simulink model "RC_Demo_C2000_Control_Unit"  (R2019b)
settings: Solver=FixedStepDiscrete  StartTime=0.0  StopTime=inf  FixedStep=0.01  RelTol=1e-3  EnableMultiTasking=on
undefined symbols (not defined in the file): Down, GPTRIP1SEL, GPTRIP2SEL, TZ1, TZ2, Up
libraries: c280xlib x11, canmsglib x6, dspstat3 x2, c2802xlib x2, c2837xDlib x1, c2000lib x1
settings Model: ExtModeTrigDuration=8  Creator=The MathWorks, Inc.  LastModifiedBy=bhisma
settings DataIOCC: LimitDataPoints=on  SaveFormat=Array  SaveOutput=off  SaveTime=off  ReturnWorkspaceOutputs=off
settings OptimizationCC: DefaultUnderspecifiedDataType=single  PassReuseOutputArgsAs=Individual arguments  ExpressionDepthLimit=2147483647  MaxStackSize=512  EfficientTunableParamExpr=on
settings DebuggingCC: UnderspecifiedInitializationDetection=Classic  MergeDetectMultiDrivingBlocksExec=none  SolverPrmCheckMsg=warning  MultiTaskDSMMsg=none  TasksWithSamePriorityMsg=none  ParameterPrecisionLossMsg=none  ParameterTunabilityLossMsg=error  FcnCallInpInsideContextMsg=warning  StateNameClashWarn=warning  SFUnexpectedBacktrackingDiag=warning  SFNoUnconditionalDefaultTransitionDiag=warning  SFExecutionAtInitializationDiag=none  ArithmeticOperatorsInVariantConditions=warning
settings HardwareCC: ProdBitPerChar=16  ProdBitPerInt=16  ProdBitPerPointer=32  ProdBitPerSizeT=32  ProdBitPerPtrDiffT=32  ProdLargestAtomicInteger=Integer  ProdLargestAtomicFloat=None  ProdWordSize=16  ProdLongLongMode=on  ProdHWDeviceType=Texas Instruments->C2000
settings ModelReferenceCC: PropagateSignalLabelsOutOfModel=off
settings SFSimCC: SimUseLocalCustomCode=off  CustomCodeUndefinedFunction=UseInterfaceOnly
settings RTWCC: SystemTargetFile=ert.tlc  HardwareBoard=TI Delfino F2837xD  TLCOptions=-aInlineSetEventsForThisBaseRateFcn=TLC_FALSE -aSuppressMultiTaskScheduler=TLC_FALSE -aRateBasedStepFcn=1  TemplateMakefile=ert_default_tmf  GenerateReport=on  RTWUseLocalCustomCode=off  Toolchain=Texas Instruments Code Composer Studio v6 (C2000)  IncludeHyperlinkInReport=on  LaunchReport=on  GenerateTraceInfo=on  GenerateTraceReport=on  GenerateTraceReportSl=on  GenerateTraceReportSf=on  GenerateTraceReportEml=on
settings CodeAppCC: ForceParamTrailComments=on  IgnoreCustomStorageClasses=off  OperatorAnnotations=on  SimulinkDataObjDesc=on  SFDataObjDesc=on  MATLABFcnDesc=on  InsertBlockDesc=on  StateflowObjectComments=on  MATLABSourceComments=on
settings ERTTargetCC: CodeReplacementLibrary=TI C28x
settings ConfigComp: CovMetricSettings=dw  CovHtmlReporting=on  CovSaveCumulativeToWorkspaceVar=on  CovSaveSingleToWorkspaceVar=on  CovExternalEMLEnable=off
settings TargetHardwareResources: Description=Target Hardware Resources Component

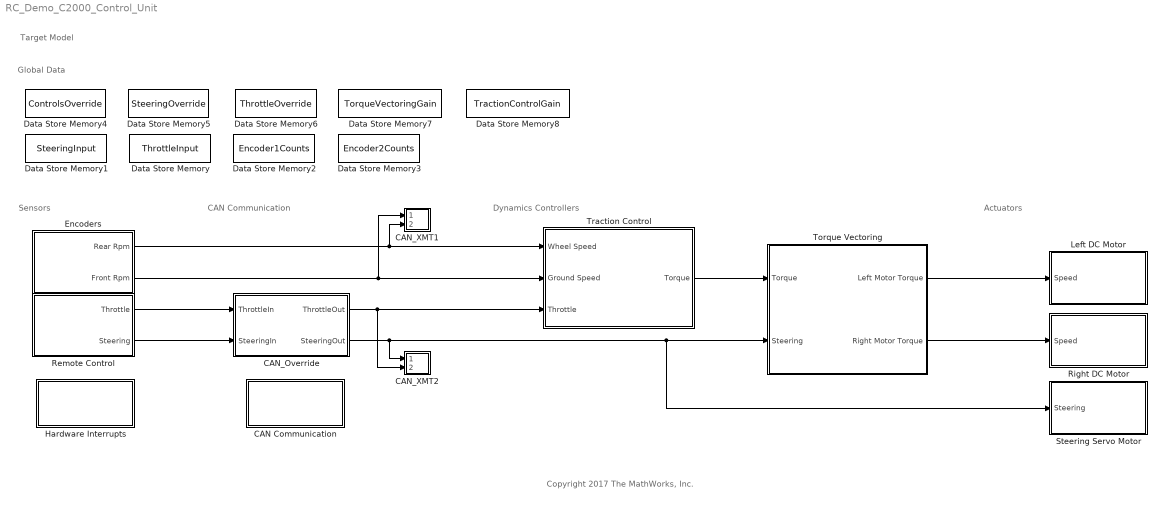
== system RC_Demo_C2000_Control_Unit ==
  note: Actuators
  note: Dynamics Controllers
  note: CAN Communication
  note: Sensors
  note: Global Data
  note: Target Model
  note: Copyright 2017 The MathWorks, Inc.
  CAN Communication : Subsystem
  CAN_Override : Subsystem
  CAN_XMT1 : Subsystem
  CAN_XMT2 : Subsystem
  Data Store Memory : DataStoreMemory  DataStoreName=ThrottleInput  ReadBeforeWriteMsg=warning  WriteAfterWriteMsg=warning  WriteAfterReadMsg=warning  ShowAdditionalParam=off
  Data Store Memory1 : DataStoreMemory  DataStoreName=SteeringInput  ReadBeforeWriteMsg=warning  WriteAfterWriteMsg=warning  WriteAfterReadMsg=warning  ShowAdditionalParam=off
  Data Store Memory2 : DataStoreMemory  DataStoreName=Encoder1Counts  ReadBeforeWriteMsg=warning  WriteAfterWriteMsg=warning  WriteAfterReadMsg=warning  ShowAdditionalParam=off  OutDataTypeStr=double
  Data Store Memory3 : DataStoreMemory  DataStoreName=Encoder2Counts  ReadBeforeWriteMsg=warning  WriteAfterWriteMsg=warning  WriteAfterReadMsg=warning  ShowAdditionalParam=off  OutDataTypeStr=double
  Data Store Memory4 : DataStoreMemory  DataStoreName=ControlsOverride  ReadBeforeWriteMsg=warning  WriteAfterWriteMsg=warning  WriteAfterReadMsg=warning  ShowAdditionalParam=off  OutDataTypeStr=int8
  Data Store Memory5 : DataStoreMemory  DataStoreName=SteeringOverride  ReadBeforeWriteMsg=warning  WriteAfterWriteMsg=warning  WriteAfterReadMsg=warning  ShowAdditionalParam=off  OutDataTypeStr=double
  Data Store Memory6 : DataStoreMemory  DataStoreName=ThrottleOverride  ReadBeforeWriteMsg=warning  WriteAfterWriteMsg=warning  WriteAfterReadMsg=warning  ShowAdditionalParam=off  OutDataTypeStr=double
  Data Store Memory7 : DataStoreMemory  DataStoreName=TorqueVectoringGain  ReadBeforeWriteMsg=warning  WriteAfterWriteMsg=warning  WriteAfterReadMsg=warning  ShowAdditionalParam=off  OutDataTypeStr=double
  Data Store Memory8 : DataStoreMemory  DataStoreName=TractionControlGain  ReadBeforeWriteMsg=warning  WriteAfterWriteMsg=warning  WriteAfterReadMsg=warning  ShowAdditionalParam=off  OutDataTypeStr=double
  Encoders : Subsystem
      mask Display:
      | pic = imread('Icons/WheelIcon.jpg');
      | pos = get_param(gcb, 'Position');
      | width  = pos(3) - pos(1);
      | height = pos(4) - pos(2);
      | x = (width - 40 - 20)/2;
      | y = (height - 40)/2;
      | image(pic,[x y 40 40]);
      | port_label('output',1,'Rear Rpm');
      | port_label('output',2,'Front Rpm');
  Hardware Interrupts : Subsystem
  Left DC Motor : Subsystem
      mask Display:
      | pic=imread('Icons/dcMotor.png');
      | image(pic,[(1-58/110)/2 (1-35/60)/2 58/110 35/60]);
      | color('blue');
      | text(0.99, 0.90, 'CAN RC Demo', 'horizontalAlignment', 'right');
  Remote Control : Subsystem
      mask Display:
      | pic = imread('Icons/SteeringIcon.png');
      | pos = get_param(gcb, 'Position');
      | width  = pos(3) - pos(1);
      | height = pos(4) - pos(2);
      | x = (width - 40 - 30)/2;
      | y = (height - 40)/2;
      | image(pic,[x y 45 40]);
      | port_label('output',1,'Throttle');
      | port_label('output',2,'Steering');
  Right DC Motor : Subsystem
      mask Display:
      | pic=imread('Icons/dcMotor.png');
      | image(pic,[(1-58/110)/2 (1-35/60)/2 58/110 35/60]);
      | color('blue');
      | text(0.99, 0.90, 'CAN RC Demo', 'horizontalAlignment', 'right');
  Steering Servo Motor : Subsystem
      mask Display:
      | pic=imread('Icons/servowrite.png');
      | image(pic,[0.32 0.23 0.35 0.53]);
      | color('blue');
      | text(0.99, 0.90, 'CAN RC Demo', 'horizontalAlignment', 'right');
  Torque Vectoring : Subsystem
      mask Display:
      | pic = imread('Icons/TVIcon.png');
      | pos = get_param(gcb, 'Position');
      | width  = pos(3) - pos(1);
      | height = pos(4) - pos(2);
      | x = (width  - 100)/2;
      | y = (height + 220)/10;
      | image(pic,[x y 80 80]);
      | port_label('output',1,'Left Motor Torque');
      | port_label('output',2,'Right Motor Torque');
      | port_label('input',1,'Torque');
      | port_label('input',2,'Steering');
  Traction Control : Subsystem
      mask Display:
      | pic = imread('Icons/TCIcon.png');
      | pos = get_param(gcb, 'Position');
      | width  = pos(3) - pos(1);
      | height = pos(4) - pos(2);
      | x = (width  - 40)/2;
      | y = (height - 80)/2;
      | image(pic,[x y 70 80]);
      | port_label('output',1,'Torque');
      | port_label('input',1,'Wheel Speed');
      | port_label('input',2,'Ground Speed');
      | port_label('input',3,'Throttle');
  wires:
  Traction Control/1(Torque) -> Torque Vectoring/1(Torque)
  CAN_Override/1(ThrottleOut) -> Traction Control/3(Throttle), CAN_XMT2/2(In2)
  CAN_Override/2(SteeringOut) -> CAN_XMT2/1(In1), Torque Vectoring/2(Steering), Steering Servo Motor/1(Steering)
  Torque Vectoring/1(Left Motor Torque) -> Left DC Motor/1(Speed)
  Torque Vectoring/2(Right Motor Torque) -> Right DC Motor/1(Speed)
  Encoders/1(Rear Rpm) -> Traction Control/1(Wheel Speed), CAN_XMT1/2(In2)
  Encoders/2(Front Rpm) -> Traction Control/2(Ground Speed), CAN_XMT1/1(In1)
  Remote Control/1(Throttle) -> CAN_Override/1(ThrottleIn)
  Remote Control/2(Steering) -> CAN_Override/2(SteeringIn)

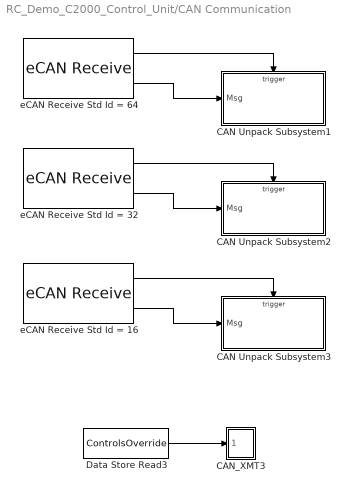
== system RC_Demo_C2000_Control_Unit/CAN Communication ==
  CAN Unpack Subsystem1 : Subsystem  TreatAsAtomicUnit=on
  CAN Unpack Subsystem2 : Subsystem  TreatAsAtomicUnit=on
  CAN Unpack Subsystem3 : Subsystem  TreatAsAtomicUnit=on
  CAN_XMT3 : Subsystem
  Data Store Read3 : DataStoreRead  DataStoreName=ControlsOverride
  eCAN Receive Std Id = 16 : c280xlib/eCAN Receive  chipFamily=C280x  useModule=eCAN_B  mailboxNo=17  messageID=16  messageType=Standard (11-bit identifier)  sampleTime=0.01  dataType=CAN_MESSAGE_TYPE  initValue=0  outputMessageLength=off  outputMessageTimeStamp=off  postInterrupt=off  interruptLine=0
      settings: SourceProductName=Embedded Coder Support Package for Texas Instruments C2000 Processors  SourceProductBaseCode=TIC2000
  eCAN Receive Std Id = 32 : c280xlib/eCAN Receive  chipFamily=C280x  useModule=eCAN_B  mailboxNo=16  messageID=32  messageType=Standard (11-bit identifier)  sampleTime=0.01  dataType=CAN_MESSAGE_TYPE  initValue=0  outputMessageLength=off  outputMessageTimeStamp=off  postInterrupt=off  interruptLine=0
      settings: SourceProductName=Embedded Coder Support Package for Texas Instruments C2000 Processors  SourceProductBaseCode=TIC2000
  eCAN Receive Std Id = 64 : c280xlib/eCAN Receive  chipFamily=C280x  useModule=eCAN_B  mailboxNo=15  messageID=64  messageType=Standard (11-bit identifier)  sampleTime=0.01  dataType=CAN_MESSAGE_TYPE  initValue=0  outputMessageLength=off  outputMessageTimeStamp=off  postInterrupt=off  interruptLine=0
      settings: SourceProductName=Embedded Coder Support Package for Texas Instruments C2000 Processors  SourceProductBaseCode=TIC2000
  wires:
  eCAN Receive Std Id = 64/1 -> CAN Unpack Subsystem1/Trigger
  eCAN Receive Std Id = 64/2 -> CAN Unpack Subsystem1/1(Msg)
  eCAN Receive Std Id = 32/1 -> CAN Unpack Subsystem2/Trigger
  eCAN Receive Std Id = 32/2 -> CAN Unpack Subsystem2/1(Msg)
  Data Store Read3/1 -> CAN_XMT3/1(In1)
  eCAN Receive Std Id = 16/2 -> CAN Unpack Subsystem3/1(Msg)
  eCAN Receive Std Id = 16/1 -> CAN Unpack Subsystem3/Trigger

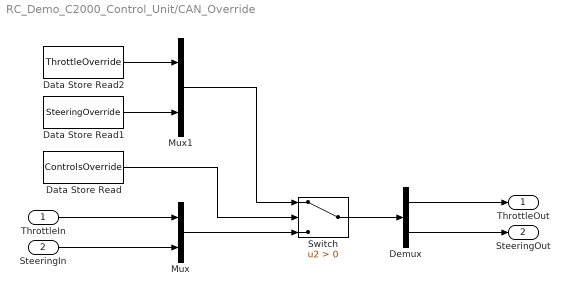
== system RC_Demo_C2000_Control_Unit/CAN_Override ==
  ThrottleIn : Inport
  SteeringIn : Inport  Port=2
  Data Store Read : DataStoreRead  DataStoreName=ControlsOverride
  Data Store Read1 : DataStoreRead  DataStoreName=SteeringOverride
  Data Store Read2 : DataStoreRead  DataStoreName=ThrottleOverride
  Demux : Demux  Outputs=2
  Mux : Mux  Inputs=2
  Mux1 : Mux  Inputs=2
  Switch : Switch  Criteria=u2 > Threshold
  ThrottleOut : Outport
  SteeringOut : Outport  Port=2
  wires:
  Data Store Read/1 -> Switch/2
  Mux1/1 -> Switch/1
  Mux/1 -> Switch/3
  Switch/1 -> Demux/1
  SteeringIn/1 -> Mux/2
  ThrottleIn/1 -> Mux/1
  Demux/1 -> ThrottleOut/1
  Demux/2 -> SteeringOut/1
  Data Store Read1/1 -> Mux1/2
  Data Store Read2/1 -> Mux1/1

== system RC_Demo_C2000_Control_Unit/CAN_XMT1 ==
  In1 : Inport
  In2 : Inport  Port=2
  CAN Pack1 : canmsglib/CAN Pack  CANdbFile=C:\Users\josea\Desktop\C2000\CAN\Vector\RCDemo.dbc  MsgList=WheelSpeeds  MsgName=WheelSpeeds  MsgIDType=Standard (11-bit identifier)  MsgIdentifier=48  MsgLength=8  SignalInfo=FrontWheelSpeed$24$32$2$3$1$0$1$0$-3.400000e+38$3.400000e+38$#RearWheelSpeed$56$32$2$3$1$0$1$0$-3.400000e+38$3.400000e+38$#  NSignals=2  StartBits=str2num('[int32(24);int32(56)]')  SignalSizes=str2num('[int32(32);int32(32)]')  ByteOrders=str2num('[int32(2);int32(2)]')  DataTypes=str2num('[int32(3);int32(3)]')  MultiplexTypes=str2num('[int32(1);int32(1)]')  MultiplexValues=str2num('[double(0);double(0)]')  Factors=str2num('[double(1);double(1)]')  Offsets=str2num('[double(0);double(0)]')  Minimums=str2num('[double(-3.400000e+38);double(-3.400000e+38)]')  Maximums=str2num('[double(3.400000e+38);double(3.400000e+38)]')  Remote=off  ApplyMinMax=off
      settings: SourceProductName=Simulink Real-Time  DataFormat=CANdb specified signals
  eCAN Transmit1 : c280xlib/eCAN Transmit  chipFamily=C280x  useModule=eCAN_B  mailboxNo=0  messageID=48  messageType=Standard (11-bit identifier)  enableBlockingMode=off  postInterrupt=off  interruptLine=0
      settings: SourceProductName=Embedded Coder Support Package for Texas Instruments C2000 Processors  SourceProductBaseCode=TIC2000
  wires:
  CAN Pack1/1 -> eCAN Transmit1/1
  In1/1 -> CAN Pack1/1
  In2/1 -> CAN Pack1/2

== system RC_Demo_C2000_Control_Unit/CAN_XMT2 ==
  In1 : Inport
  In2 : Inport  Port=2
  CAN Pack2 : canmsglib/CAN Pack  CANdbFile=C:\Users\josea\Desktop\C2000\CAN\Vector\RCDemo.dbc  MsgList=DriverControlsFromCar  MsgName=DriverControlsFromCar  MsgIDType=Standard (11-bit identifier)  MsgIdentifier=33  MsgLength=8  SignalInfo=SteeringInput$32$32$1$3$1$0$1$0$-3.400000e+38$3.400000e+38$#ThrottleInput$0$32$1$3$1$0$1$0$-3.400000e+38$3.400000e+38$#  NSignals=2  StartBits=str2num('[int32(32);int32(0)]')  SignalSizes=str2num('[int32(32);int32(32)]')  ByteOrders=str2num('[int32(1);int32(1)]')  DataTypes=str2num('[int32(3);int32(3)]')  MultiplexTypes=str2num('[int32(1);int32(1)]')  MultiplexValues=str2num('[double(0);double(0)]')  Factors=str2num('[double(1);double(1)]')  Offsets=str2num('[double(0);double(0)]')  Minimums=str2num('[double(-3.400000e+38);double(-3.400000e+38)]')  Maximums=str2num('[double(3.400000e+38);double(3.400000e+38)]')  Remote=off  ApplyMinMax=off
      settings: SourceProductName=Simulink Real-Time  DataFormat=CANdb specified signals
  eCAN Transmit2 : c280xlib/eCAN Transmit  chipFamily=C280x  useModule=eCAN_B  mailboxNo=1  messageID=33  messageType=Standard (11-bit identifier)  enableBlockingMode=off  postInterrupt=off  interruptLine=0
      settings: SourceProductName=Embedded Coder Support Package for Texas Instruments C2000 Processors  SourceProductBaseCode=TIC2000
  wires:
  CAN Pack2/1 -> eCAN Transmit2/1
  In2/1 -> CAN Pack2/2
  In1/1 -> CAN Pack2/1

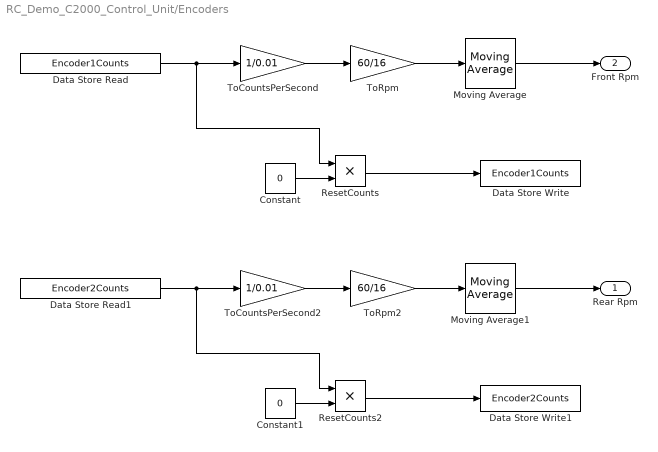
== system RC_Demo_C2000_Control_Unit/Encoders ==
  Constant : Constant  Value=0
  Constant1 : Constant  Value=0
  Data Store Read : DataStoreRead  Priority=1  DataStoreName=Encoder1Counts
  Data Store Read1 : DataStoreRead  Priority=1  DataStoreName=Encoder2Counts
  Data Store Write : DataStoreWrite  DataStoreName=Encoder1Counts
  Data Store Write1 : DataStoreWrite  DataStoreName=Encoder2Counts
  Moving Average : dspstat3/Moving Average  Method=Sliding window  SpecifyWindowLength=on  WindowLength=10  ForgettingFactor=0.9  SimulateUsing=Code generation
  Moving Average1 : dspstat3/Moving Average  Method=Sliding window  SpecifyWindowLength=on  WindowLength=10  ForgettingFactor=0.9  SimulateUsing=Code generation
  ResetCounts : Product  Inputs=**
  ResetCounts2 : Product  Inputs=**
  ToCountsPerSecond : Gain  Gain=1/0.01
  ToCountsPerSecond2 : Gain  Gain=1/0.01
  ToRpm : Gain  Gain=60/16
  ToRpm2 : Gain  Gain=60/16
  Rear Rpm : Outport
  Front Rpm : Outport  Port=2
  wires:
  Moving Average1/1 -> Rear Rpm/1
  Data Store Read1/1 -> ResetCounts2/1, ToCountsPerSecond2/1
  ToCountsPerSecond2/1 -> ToRpm2/1
  ToRpm2/1 -> Moving Average1/1
  Constant1/1 -> ResetCounts2/2
  ResetCounts2/1 -> Data Store Write1/1
  ResetCounts/1 -> Data Store Write/1
  Constant/1 -> ResetCounts/2
  ToRpm/1 -> Moving Average/1
  ToCountsPerSecond/1 -> ToRpm/1
  Data Store Read/1 -> ToCountsPerSecond/1, ResetCounts/1
  Moving Average/1 -> Front Rpm/1

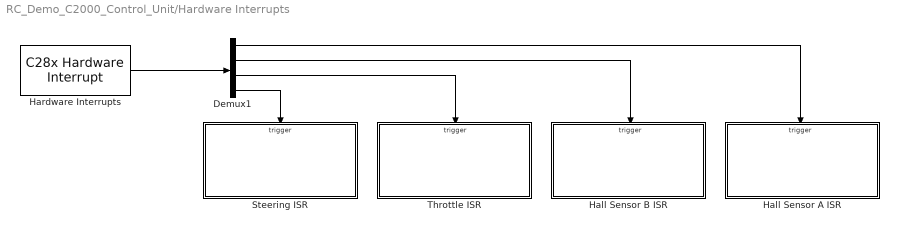
== system RC_Demo_C2000_Control_Unit/Hardware Interrupts ==
  Demux1 : Demux
  Hall Sensor A ISR : Subsystem  TreatAsAtomicUnit=on
  Hall Sensor B ISR : Subsystem  TreatAsAtomicUnit=on
  Hardware Interrupts : c2000lib/Scheduling/C28x Hardware Interrupt  irqnumbers=[4 4 4 4]  pienumbers=[1 2 3 4]  irqpriorities=[25 25 2 2]  irqpreempts=[1 1 0 0]  showinput=off  dspchiptype=C280X
      settings: SourceProductName=Embedded Coder Support Package for Texas Instruments C2000 Processors  SourceProductBaseCode=TIC2000
  Steering ISR : Subsystem  TreatAsAtomicUnit=on
  Throttle ISR : Subsystem  TreatAsAtomicUnit=on
  wires:
  Hardware Interrupts/1 -> Demux1/1
  Demux1/1 -> Hall Sensor A ISR/Trigger
  Demux1/4 -> Steering ISR/Trigger
  Demux1/3 -> Throttle ISR/Trigger
  Demux1/2 -> Hall Sensor B ISR/Trigger

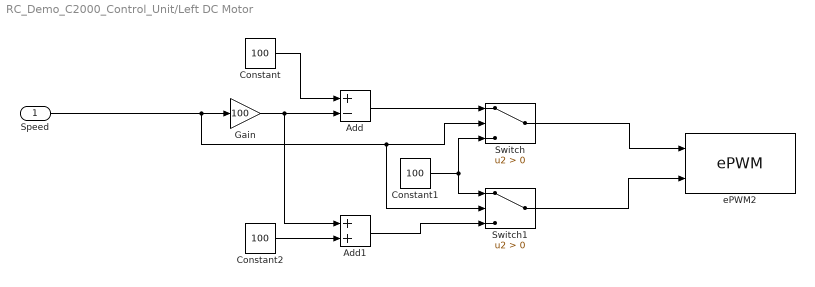
== system RC_Demo_C2000_Control_Unit/Left DC Motor ==
  Speed : Inport
  Add : Sum  Inputs=+-
  Add1 : Sum
  Constant : Constant  Value=100
  Constant1 : Constant  Value=100
  Constant2 : Constant  Value=100
  Gain : Gain  Gain=100
  Switch : Switch  Criteria=u2 > Threshold
  Switch1 : Switch  Criteria=u2 > Threshold
  ePWM2 : c2802xlib/ePWM  useModule=ePWM2  ePWMxLINKTBPRD=Not Linked  periodUnits=Clock cycles  timerSource=Specify via dialog  timerPeriod_clk=4000  timerPeriod_sec=0.02  tbshadow=Counter equals to zero  countingMode=Up-Down  phaseActiveEnable=Disable  phaseDirection=Count down after sync  phaseActive=0  synchronizationEnable=off  dcaevt1Sync=off  dcbevt1Sync=off  synchronizationOption=Disable  clockPrescale=1  HSclockPrescale=1  enswap=off  ePWMxAStatus=on  ePWMxAactionLogic1=Do nothing  ePWMxAactionLogic2=Do nothing  ePWMxAactionLogic3=Set  ePWMxAactionLogic4=Clear  ePWMxAactionLogic5=Do nothing  ePWMxAactionLogic6=Do nothing  ePWMxALoadMode=Load on counter equals to zero (CTR=Zero)  ePWMxACSFenable=off  ePWMxACSFvalue=Forcing disable  ePWMxASFreload=Zero  ePWMxBStatus=on  ePWMxBactionLogic1=Do nothing  ePWMxBactionLogic2=Do nothing  ePWMxBactionLogic3=Do nothing  ePWMxBactionLogic4=Do nothing  ePWMxBactionLogic5=Set  ePWMxBactionLogic6=Clear  ePWMxBLoadMode=Load on counter equals to zero (CTR=Zero)  ePWMxBCSFenable=off  ePWMxBCSFvalue=Forcing disable  ePWMxBSFreload=Zero  ePWNxBOutWay=off  ePWMxLINKCMPA=Not Linked  CMPAUnits=Percentages  CMPASource=Input port  CMPAValue_per=0  CMPAValue_clk=5000  enCMPAshadow=Counter equals to zero  ePWMxLINKCMPB=Not Linked  CMPBUnits=Percentages  CMPBSource=Input port  CMPBValue_per=0  CMPBValue_clk=0  enCMPBshadow=Counter equals to zero  ePWMxLINKCMPC=Not Linked  CMPCUnits=Clock cycles  CMPCSource=Specify via dialog  CMPCValue_per=50  CMPCValue_clk=0  enCMPCshadow=Counter equals to zero  ePWMxLINKCMPD=Not Linked  CMPDUnits=Clock cycles  CMPDSource=Specify via dialog  CMPDValue_per=50  CMPDValue_clk=0  enCMPDshadow=Counter equals to zero  enableDBePWMxA=off  enableDBePWMxB=off  enhalfcycle=off  DBpolarity=Active high (AH)  DBedgeDelay=Positive  DBSource_ePWMxA=ePWMxA  DBSource_ePWMxB=ePWMxA  DBperiodSource=Specify via dialog  REDperiod=0  FEDperiod=0  adcstartModuleA=on  adcrequestEventA=First event  adcstartEventA=Digital Compare Module A Event 1 start of conversion (DCAEVT1.soc)  adcstartEventA_type2=Counter equals to period (CTR=PRD)  adcstartModuleB=on  adcrequestEventB=First event  adcstartEventB=Counter equals to zero (CTR=Zero)  adcstartEventB_type2=Counter equals to zero (CTR=Zero)  intEn=off  intPrd=First event  intSel=Counter equals to zero (CTR=Zero)  intSel_type2=Counter equals to zero (CTR=Zero)  hrpe=off  enHRPWM=off  HRPWM_LoadMode=Counter equals to period (CTR=PRD)  HRPWM_CTLMode=Duty or Period control mode  HRPWM_EDGMode=Both edge  hrpeb=off  enHRPWMB=off  HRPWM_LoadModeB=Counter equals to zero (CTR=ZERO)  HRPWM_CTLModeB=Duty or Period control mode  HRPWM_EDGModeB=Both edge  enSFO=on  enautoconv=on  chopperEnable=off  chopperFrequency=1  chopperFirstwidth=1  chopperDuty=12.5%  tripZonesource=Specify via dialog  tzselOSHT1=off  tzselOSHT2=off  tzselOSHT3=off  tzselOSHDCAEV1=off  tzselOSHDCBEV1=off  tzselCBC1=off  tzselCBC2=off  tzselCBC3=off  tzselCBCDCAEV2=off  tzselCBCDCBEV2=off  tzselOSHT4=off  tzselOSHT5=off  tzselOSHT6=off  tzselCBC4=off  tzselCBC5=off  tzselCBC6=off  enTzOstIntr=off  enTzCbcIntr=off  enTzDCAEVT1Intr=off  enTzDCAEVT2Intr=off  enTzDCBEVT1Intr=off  enTzDCBEVT2Intr=off  ePWMxAforced=No action  ePWMxBforced=No action  DCAEVT1forced=No action  DCBEVT1forced=No action  DCAEVT2forced=No action  DCBEVT2forced=No action  dcah=Trip Zone 1 input (TZ1)  dcal=Trip Zone 2 input (TZ2)  dcbh=Trip Zone 1 input (TZ1)  dcbl=Trip Zone 2 input (TZ2)  dcah_type2=GPTRIP1SEL/(TZ1)  dcal_type2=GPTRIP2SEL/(TZ2)  dcbh_type2=GPTRIP1SEL/(TZ1)  dcbl_type2=GPTRIP2SEL/(TZ2)  gendcaevt1=Event disabled  gendcaevt2=Event disabled  gendcbevt1=Event disabled  gendcbevt2=Event disabled  dcaevt1src=DCAEVT1 with sync  dcaevt2src=DCAEVT2 with sync  dcbevt1src=DCBEVT1 with sync  dcbevt2src=DCBEVT2 with sync  pulsesel=Counter equals to zero (CTR=Zero)  blankinv=off  blankoffset=0  blankwidth=0  evsrcsel=Filtered version of DCAEVT1 (DCAEVT1FILT)  encape=off  PwmType=C2000_Type4
      settings: SourceProductName=Embedded Coder Support Package for Texas Instruments C2000 Processors
  wires:
  Switch/1 -> ePWM2/1
  Constant2/1 -> Add1/2
  Add/1 -> Switch/1
  Add1/1 -> Switch1/3
  Constant1/1 -> Switch/3, Switch1/1
  Constant/1 -> Add/1
  Gain/1 -> Add1/1, Add/2
  Speed/1 -> Switch1/2, Switch/2, Gain/1
  Switch1/1 -> ePWM2/2

== system RC_Demo_C2000_Control_Unit/Remote Control ==
  Data Store Read : DataStoreRead  DataStoreName=ThrottleInput
  Data Store Read1 : DataStoreRead  DataStoreName=SteeringInput
  Throttle : Outport
  Steering : Outport  Port=2
  wires:
  Data Store Read/1 -> Throttle/1
  Data Store Read1/1 -> Steering/1

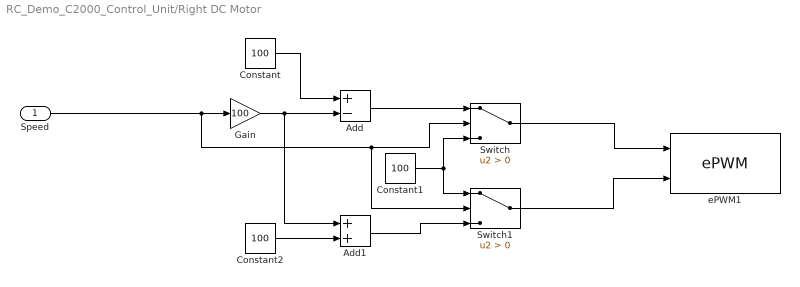
== system RC_Demo_C2000_Control_Unit/Right DC Motor ==
  Speed : Inport
  Add : Sum  Inputs=+-
  Add1 : Sum
  Constant : Constant  Value=100
  Constant1 : Constant  Value=100
  Constant2 : Constant  Value=100
  Gain : Gain  Gain=100
  Switch : Switch  Criteria=u2 > Threshold
  Switch1 : Switch  Criteria=u2 > Threshold
  ePWM1 : c2802xlib/ePWM  useModule=ePWM1  ePWMxLINKTBPRD=Not Linked  periodUnits=Clock cycles  timerSource=Specify via dialog  timerPeriod_clk=4000  timerPeriod_sec=0.02  tbshadow=Counter equals to zero  countingMode=Up-Down  phaseActiveEnable=Disable  phaseDirection=Count down after sync  phaseActive=0  synchronizationEnable=off  dcaevt1Sync=off  dcbevt1Sync=off  synchronizationOption=Disable  clockPrescale=1  HSclockPrescale=1  enswap=off  ePWMxAStatus=on  ePWMxAactionLogic1=Do nothing  ePWMxAactionLogic2=Do nothing  ePWMxAactionLogic3=Set  ePWMxAactionLogic4=Clear  ePWMxAactionLogic5=Do nothing  ePWMxAactionLogic6=Do nothing  ePWMxALoadMode=Load on counter equals to zero (CTR=Zero)  ePWMxACSFenable=off  ePWMxACSFvalue=Forcing disable  ePWMxASFreload=Zero  ePWMxBStatus=on  ePWMxBactionLogic1=Do nothing  ePWMxBactionLogic2=Do nothing  ePWMxBactionLogic3=Do nothing  ePWMxBactionLogic4=Do nothing  ePWMxBactionLogic5=Set  ePWMxBactionLogic6=Clear  ePWMxBLoadMode=Load on counter equals to zero (CTR=Zero)  ePWMxBCSFenable=off  ePWMxBCSFvalue=Forcing disable  ePWMxBSFreload=Zero  ePWNxBOutWay=off  ePWMxLINKCMPA=Not Linked  CMPAUnits=Percentages  CMPASource=Input port  CMPAValue_per=0  CMPAValue_clk=5000  enCMPAshadow=Counter equals to zero  ePWMxLINKCMPB=Not Linked  CMPBUnits=Percentages  CMPBSource=Input port  CMPBValue_per=0  CMPBValue_clk=0  enCMPBshadow=Counter equals to zero  ePWMxLINKCMPC=Not Linked  CMPCUnits=Clock cycles  CMPCSource=Specify via dialog  CMPCValue_per=50  CMPCValue_clk=0  enCMPCshadow=Counter equals to zero  ePWMxLINKCMPD=Not Linked  CMPDUnits=Clock cycles  CMPDSource=Specify via dialog  CMPDValue_per=50  CMPDValue_clk=0  enCMPDshadow=Counter equals to zero  enableDBePWMxA=off  enableDBePWMxB=off  enhalfcycle=off  DBpolarity=Active high (AH)  DBedgeDelay=Positive  DBSource_ePWMxA=ePWMxA  DBSource_ePWMxB=ePWMxA  DBperiodSource=Specify via dialog  REDperiod=0  FEDperiod=0  adcstartModuleA=on  adcrequestEventA=First event  adcstartEventA=Digital Compare Module A Event 1 start of conversion (DCAEVT1.soc)  adcstartEventA_type2=Counter equals to period (CTR=PRD)  adcstartModuleB=on  adcrequestEventB=First event  adcstartEventB=Counter equals to zero (CTR=Zero)  adcstartEventB_type2=Counter equals to zero (CTR=Zero)  intEn=off  intPrd=First event  intSel=Counter equals to zero (CTR=Zero)  intSel_type2=Counter equals to zero (CTR=Zero)  hrpe=off  enHRPWM=off  HRPWM_LoadMode=Counter equals to period (CTR=PRD)  HRPWM_CTLMode=Duty or Period control mode  HRPWM_EDGMode=Both edge  hrpeb=off  enHRPWMB=off  HRPWM_LoadModeB=Counter equals to zero (CTR=ZERO)  HRPWM_CTLModeB=Duty or Period control mode  HRPWM_EDGModeB=Both edge  enSFO=on  enautoconv=on  chopperEnable=off  chopperFrequency=1  chopperFirstwidth=1  chopperDuty=12.5%  tripZonesource=Specify via dialog  tzselOSHT1=off  tzselOSHT2=off  tzselOSHT3=off  tzselOSHDCAEV1=off  tzselOSHDCBEV1=off  tzselCBC1=off  tzselCBC2=off  tzselCBC3=off  tzselCBCDCAEV2=off  tzselCBCDCBEV2=off  tzselOSHT4=off  tzselOSHT5=off  tzselOSHT6=off  tzselCBC4=off  tzselCBC5=off  tzselCBC6=off  enTzOstIntr=off  enTzCbcIntr=off  enTzDCAEVT1Intr=off  enTzDCAEVT2Intr=off  enTzDCBEVT1Intr=off  enTzDCBEVT2Intr=off  ePWMxAforced=No action  ePWMxBforced=No action  DCAEVT1forced=No action  DCBEVT1forced=No action  DCAEVT2forced=No action  DCBEVT2forced=No action  dcah=Trip Zone 1 input (TZ1)  dcal=Trip Zone 2 input (TZ2)  dcbh=Trip Zone 1 input (TZ1)  dcbl=Trip Zone 2 input (TZ2)  dcah_type2=GPTRIP1SEL/(TZ1)  dcal_type2=GPTRIP2SEL/(TZ2)  dcbh_type2=GPTRIP1SEL/(TZ1)  dcbl_type2=GPTRIP2SEL/(TZ2)  gendcaevt1=Event disabled  gendcaevt2=Event disabled  gendcbevt1=Event disabled  gendcbevt2=Event disabled  dcaevt1src=DCAEVT1 with sync  dcaevt2src=DCAEVT2 with sync  dcbevt1src=DCBEVT1 with sync  dcbevt2src=DCBEVT2 with sync  pulsesel=Counter equals to zero (CTR=Zero)  blankinv=off  blankoffset=0  blankwidth=0  evsrcsel=Filtered version of DCAEVT1 (DCAEVT1FILT)  encape=off  PwmType=C2000_Type4
      settings: SourceProductName=Embedded Coder Support Package for Texas Instruments C2000 Processors
  wires:
  Switch1/1 -> ePWM1/2
  Speed/1 -> Gain/1, Switch1/2, Switch/2
  Gain/1 -> Add/2, Add1/1
  Constant/1 -> Add/1
  Constant1/1 -> Switch1/1, Switch/3
  Add1/1 -> Switch1/3
  Add/1 -> Switch/1
  Constant2/1 -> Add1/2
  Switch/1 -> ePWM1/1

== system RC_Demo_C2000_Control_Unit/Steering Servo Motor ==
  Steering : Inport
  Add : Sum
  Offset : Constant  Value=6.25
  ToPercentDutyCycle : Gain  Gain=1.25
  eCAP5 : c280xlib/eCAP  operatingMode=APWM  selectCAPx=eCAP5  offsetValue=0  counterSynIn=off  enableCounter=off  syncOutput=Disabled  sampleTime=-1  eventPrescaler=0  selectMode=Continuous  enableOneShot=off  stopValue=Capture Event 2  resetEv1Ts=off  ev1Polarity=Falling Edge  resetEv2Ts=on  ev2Polarity=Rising Edge  resetEv3Ts=off  ev3Polarity=Rising Edge  resetEv4Ts=on  ev4Polarity=Rising Edge  tSCntrDataType=uint32  capEvFlag=off  capFlagDataType=uint16  overFlowFlag=off  overFlowFlagDataType=uint16  periodUnit=Seconds  periodSource=Specify via dialog  waveformPeriod=0.02  dutyUnit=Percentages  dutySource=Input port  dutyCycle=7.5  outputPolarity=Active High  enableCEVT1Int=off  enableCEVT2Int=on  enableCEVT3Int=off  enableCEVT4Int=on  enableCTROVFInt=off  enablePRDInt=off  enableCMPInt=off
      settings: SourceProductName=Embedded Coder Support Package for Texas Instruments C2000 Processors  SourceProductBaseCode=TIC2000
  wires:
  Steering/1 -> ToPercentDutyCycle/1
  ToPercentDutyCycle/1 -> Add/1
  Offset/1 -> Add/2
  Add/1 -> eCAP5/1

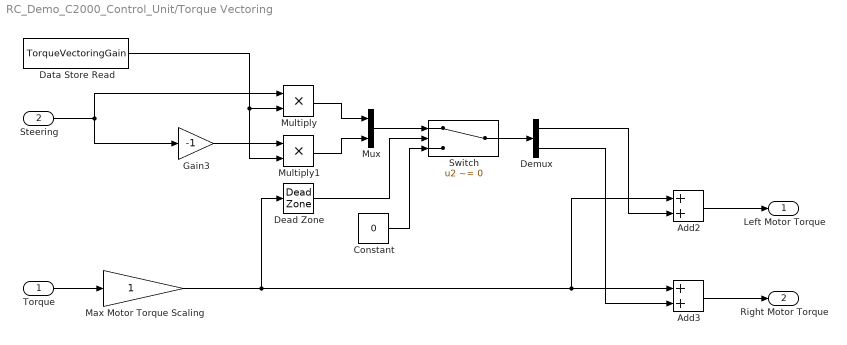
== system RC_Demo_C2000_Control_Unit/Torque Vectoring ==
  Torque : Inport
  Steering : Inport  Port=2
  Add2 : Sum
  Add3 : Sum
  Constant : Constant  Value=0
  Data Store Read : DataStoreRead  DataStoreName=TorqueVectoringGain
  Dead Zone : DeadZone  LowerValue=-0.05  UpperValue=0.05  SaturateOnIntegerOverflow=on
  Demux : Demux  Outputs=2
  Gain3 : Gain  Gain=-1
  Max Motor Torque Scaling : Gain
  Multiply : Product  Inputs=**
  Multiply1 : Product  Inputs=**
  Mux : Mux  Inputs=2
  Switch : Switch  Criteria=u2 ~= 0  Threshold=0.05
  Left Motor Torque : Outport
  Right Motor Torque : Outport  Port=2
  wires:
  Gain3/1 -> Multiply1/1
  Add3/1 -> Right Motor Torque/1
  Torque/1 -> Max Motor Torque Scaling/1
  Steering/1 -> Gain3/1, Multiply/1
  Max Motor Torque Scaling/1 -> Dead Zone/1, Add2/1, Add3/1
  Add2/1 -> Left Motor Torque/1
  Data Store Read/1 -> Multiply1/2, Multiply/2
  Multiply/1 -> Mux/1
  Multiply1/1 -> Mux/2
  Switch/1 -> Demux/1
  Dead Zone/1 -> Switch/2
  Demux/1 -> Add2/2
  Demux/2 -> Add3/2
  Mux/1 -> Switch/1
  Constant/1 -> Switch/3

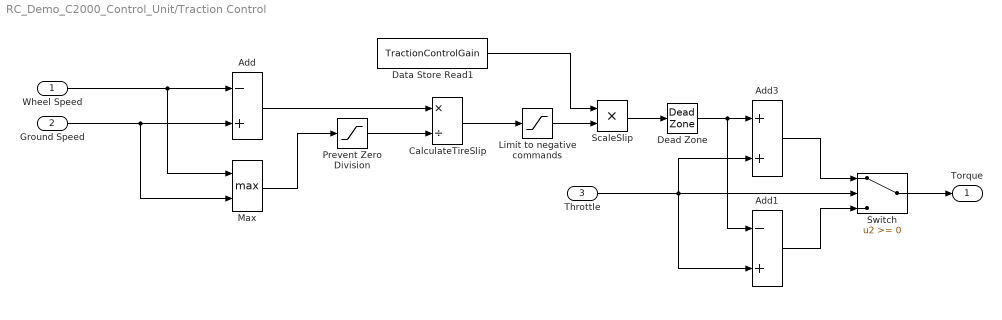
== system RC_Demo_C2000_Control_Unit/Traction Control ==
  Wheel Speed : Inport
  Ground Speed : Inport  Port=2
  Throttle : Inport  Port=3
  Add : Sum  Inputs=-+
  Add1 : Sum  Inputs=-+
  Add3 : Sum
  CalculateTireSlip : Product  Inputs=*/
  Data Store Read1 : DataStoreRead  DataStoreName=TractionControlGain
  Dead Zone : DeadZone  LowerValue=-0.05  UpperValue=0.05  SaturateOnIntegerOverflow=on
  Limit to negative commands : Saturate  UpperLimit=0  LowerLimit=-1
  Max : MinMax  Function=max  Inputs=2
  Prevent Zero Division : Saturate  UpperLimit=1000  LowerLimit=0.0001
  ScaleSlip : Product  Inputs=**
  Switch : Switch
  Torque : Outport
  wires:
  Throttle/1 -> Add3/2, Add1/2, Switch/2
  Limit to negative commands/1 -> ScaleSlip/2
  Add3/1 -> Switch/1
  Ground Speed/1 -> Max/2, Add/2
  Wheel Speed/1 -> Max/1, Add/1
  Add/1 -> CalculateTireSlip/1
  Max/1 -> Prevent Zero Division/1
  CalculateTireSlip/1 -> Limit to negative commands/1
  Prevent Zero Division/1 -> CalculateTireSlip/2
  Dead Zone/1 -> Add1/1, Add3/1
  ScaleSlip/1 -> Dead Zone/1
  Data Store Read1/1 -> ScaleSlip/1
  Switch/1 -> Torque/1
  Add1/1 -> Switch/3

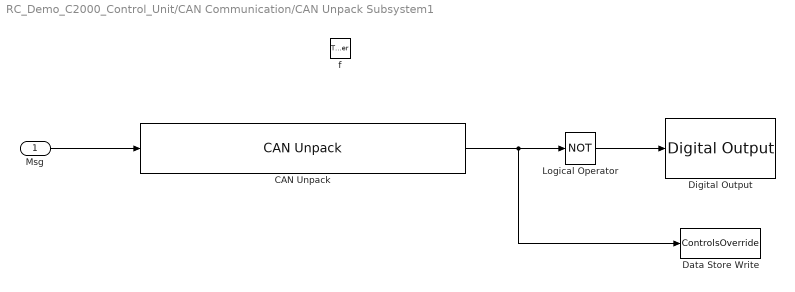
== system RC_Demo_C2000_Control_Unit/CAN Communication/CAN Unpack Subsystem1 ==
  Msg : Inport
  f : TriggerPort  TriggerType=function-call  VariantControl=Variant
  CAN Unpack : canmsglib/CAN Unpack  CANdbFile=C:\Users\josea\Desktop\C2000\CAN\Vector\RCDemo.dbc  MsgList=DriverOverrideToCar  MsgName=DriverOverrideToCar  MsgIDType=Standard (11-bit identifier)  MsgIdentifier=64  MsgLength=1  SignalInfo=DriverOverride$0$8$1$1$1$0$1$0$0$1$#  NSignals=1  IDPort=off  TimestampPort=off  ErrorPort=off  RemotePort=off  LengthPort=off  StatusPort=off  StartBits=str2num('[int32(0)]')  SignalSizes=str2num('[int32(8)]')  ByteOrders=str2num('[int32(1)]')  DataTypes=str2num('[int32(1)]')  MultiplexTypes=str2num('[int32(1)]')  MultiplexValues=str2num('[double(0)]')  Factors=str2num('[double(1)]')  Offsets=str2num('[double(0)]')  Minimums=str2num('[double(0)]')  Maximums=str2num('[double(1)]')  ApplyMinMax=off
      settings: SourceProductName=Simulink Real-Time  DataFormat=CANdb specified signals
  Data Store Write : DataStoreWrite  DataStoreName=ControlsOverride
  Digital Output : c2837xDlib/Digital Output  GPIO_Number=GPIO24~GPIO31  GPIO_Bit0=off  GPIO_BIT0_Toggle=off  GPIO_Bit1=off  GPIO_BIT1_Toggle=off  GPIO_Bit2=off  GPIO_BIT2_Toggle=off  GPIO_Bit3=off  GPIO_BIT3_Toggle=off  GPIO_Bit4=off  GPIO_BIT4_Toggle=off  GPIO_Bit5=off  GPIO_BIT5_Toggle=off  GPIO_Bit6=off  GPIO_BIT6_Toggle=off  GPIO_Bit7=on  GPIO_BIT7_Toggle=off
      settings: SourceProductName=Embedded Coder Support Package for Texas Instruments C2000 Processors  SourceProductBaseCode=TIC2000
  Logical Operator : Logic  Operator=NOT  AllPortsSameDT=off  OutDataTypeStr=boolean
  wires:
  Logical Operator/1 -> Digital Output/1
  CAN Unpack/1 -> Logical Operator/1, Data Store Write/1
  Msg/1 -> CAN Unpack/1

== system RC_Demo_C2000_Control_Unit/CAN Communication/CAN Unpack Subsystem2 ==
  Msg : Inport
  f : TriggerPort  TriggerType=function-call  VariantControl=Variant
  CAN Unpack2 : canmsglib/CAN Unpack  CANdbFile=C:\Users\josea\Desktop\C2000\CAN\Vector\RCDemo.dbc  MsgList=DriverControlsToCar  MsgName=DriverControlsToCar  MsgIDType=Standard (11-bit identifier)  MsgIdentifier=32  MsgLength=8  SignalInfo=SteeringInput$32$32$1$3$1$0$1$0$-3.400000e+38$3.400000e+38$#ThrottleInput$0$32$1$3$1$0$1$0$-3.400000e+38$3.400000e+38$#  NSignals=2  IDPort=off  TimestampPort=off  ErrorPort=off  RemotePort=off  LengthPort=off  StatusPort=off  StartBits=str2num('[int32(32);int32(0)]')  SignalSizes=str2num('[int32(32);int32(32)]')  ByteOrders=str2num('[int32(1);int32(1)]')  DataTypes=str2num('[int32(3);int32(3)]')  MultiplexTypes=str2num('[int32(1);int32(1)]')  MultiplexValues=str2num('[double(0);double(0)]')  Factors=str2num('[double(1);double(1)]')  Offsets=str2num('[double(0);double(0)]')  Minimums=str2num('[double(-3.400000e+38);double(-3.400000e+38)]')  Maximums=str2num('[double(3.400000e+38);double(3.400000e+38)]')  ApplyMinMax=off
      settings: SourceProductName=Simulink Real-Time  DataFormat=CANdb specified signals
  Data Store Write1 : DataStoreWrite  DataStoreName=SteeringOverride
  Data Store Write2 : DataStoreWrite  DataStoreName=ThrottleOverride
  wires:
  Msg/1 -> CAN Unpack2/1
  CAN Unpack2/1 -> Data Store Write1/1
  CAN Unpack2/2 -> Data Store Write2/1

== system RC_Demo_C2000_Control_Unit/CAN Communication/CAN Unpack Subsystem3 ==
  Msg : Inport
  f : TriggerPort  TriggerType=function-call  VariantControl=Variant
  CAN Unpack3 : canmsglib/CAN Unpack  CANdbFile=C:\Users\josea\Desktop\C2000\CAN\Vector\RCDemo.dbc  MsgList=DynamicsControllerGains  MsgName=DynamicsControllerGains  MsgIDType=Standard (11-bit identifier)  MsgIdentifier=16  MsgLength=8  SignalInfo=TorqueVectoringGain$0$32$1$3$1$0$1$0$0$1$#TractionControlGain$32$32$1$3$1$0$1$0$0$1$#  NSignals=2  IDPort=off  TimestampPort=off  ErrorPort=off  RemotePort=off  LengthPort=off  StatusPort=off  StartBits=str2num('[int32(0);int32(32)]')  SignalSizes=str2num('[int32(32);int32(32)]')  ByteOrders=str2num('[int32(1);int32(1)]')  DataTypes=str2num('[int32(3);int32(3)]')  MultiplexTypes=str2num('[int32(1);int32(1)]')  MultiplexValues=str2num('[double(0);double(0)]')  Factors=str2num('[double(1);double(1)]')  Offsets=str2num('[double(0);double(0)]')  Minimums=str2num('[double(0);double(0)]')  Maximums=str2num('[double(1);double(1)]')  ApplyMinMax=off
      settings: SourceProductName=Simulink Real-Time  DataFormat=CANdb specified signals
  Data Store Write1 : DataStoreWrite  DataStoreName=TorqueVectoringGain
  Data Store Write2 : DataStoreWrite  DataStoreName=TractionControlGain
  wires:
  CAN Unpack3/2 -> Data Store Write2/1
  CAN Unpack3/1 -> Data Store Write1/1
  Msg/1 -> CAN Unpack3/1

== system RC_Demo_C2000_Control_Unit/CAN Communication/CAN_XMT3 ==
  In1 : Inport
  CAN Pack3 : canmsglib/CAN Pack  CANdbFile=C:\Users\josea\Desktop\C2000\CAN\Vector\RCDemo.dbc  MsgList=DriverOverrideFromCar  MsgName=DriverOverrideFromCar  MsgIDType=Standard (11-bit identifier)  MsgIdentifier=65  MsgLength=1  SignalInfo=DriverOverride$0$8$2$1$1$0$1$0$0$1$#  NSignals=1  StartBits=str2num('[int32(0)]')  SignalSizes=str2num('[int32(8)]')  ByteOrders=str2num('[int32(2)]')  DataTypes=str2num('[int32(1)]')  MultiplexTypes=str2num('[int32(1)]')  MultiplexValues=str2num('[double(0)]')  Factors=str2num('[double(1)]')  Offsets=str2num('[double(0)]')  Minimums=str2num('[double(0)]')  Maximums=str2num('[double(1)]')  Remote=off  ApplyMinMax=off
      settings: SourceProductName=Simulink Real-Time  DataFormat=CANdb specified signals
  eCAN Transmit3 : c280xlib/eCAN Transmit  chipFamily=C280x  useModule=eCAN_B  mailboxNo=2  messageID=65  messageType=Standard (11-bit identifier)  enableBlockingMode=off  postInterrupt=off  interruptLine=0
      settings: SourceProductName=Embedded Coder Support Package for Texas Instruments C2000 Processors  SourceProductBaseCode=TIC2000
  wires:
  CAN Pack3/1 -> eCAN Transmit3/1
  In1/1 -> CAN Pack3/1

== system RC_Demo_C2000_Control_Unit/Hardware Interrupts/Hall Sensor A ISR ==
  eCAP1 Interrupt : TriggerPort  TriggerType=function-call  VariantControl=Variant
  Counter : Subsystem  TreatAsAtomicUnit=on
  Filter Glitches : If  IfExpression=u1 > 25000  ShowElse=off
  MinMax : MinMax  Function=max
  eCAP : c280xlib/eCAP  operatingMode=eCAP  selectCAPx=eCAP1  offsetValue=0  counterSynIn=off  enableCounter=off  syncOutput=Disabled  sampleTime=-1  eventPrescaler=0  selectMode=Continuous  enableOneShot=off  stopValue=Capture Event 2  resetEv1Ts=off  ev1Polarity=Falling Edge  resetEv2Ts=on  ev2Polarity=Rising Edge  resetEv3Ts=off  ev3Polarity=Rising Edge  resetEv4Ts=on  ev4Polarity=Rising Edge  tSCntrDataType=uint32  capEvFlag=off  capFlagDataType=uint16  overFlowFlag=off  overFlowFlagDataType=uint16  periodUnit=Seconds  periodSource=Specify via dialog  waveformPeriod=0.001  dutyUnit=Percentages  dutySource=Specify via dialog  dutyCycle=50  outputPolarity=Active High  enableCEVT1Int=off  enableCEVT2Int=on  enableCEVT3Int=off  enableCEVT4Int=on  enableCTROVFInt=off  enablePRDInt=off  enableCMPInt=off
      settings: SourceProductName=Embedded Coder Support Package for Texas Instruments C2000 Processors  SourceProductBaseCode=TIC2000
  wires:
  Filter Glitches/1 -> Counter/Action
  MinMax/1 -> Filter Glitches/1
  eCAP/1 -> MinMax/1

== system RC_Demo_C2000_Control_Unit/Hardware Interrupts/Hall Sensor B ISR ==
  eCAP2 Interrupt : TriggerPort  TriggerType=function-call  VariantControl=Variant
  Counter : Subsystem  TreatAsAtomicUnit=on
  Filter Glitches : If  IfExpression=u1 > 25000  ShowElse=off
  MinMax : MinMax  Function=max
  eCAP : c280xlib/eCAP  operatingMode=eCAP  selectCAPx=eCAP2  offsetValue=0  counterSynIn=off  enableCounter=off  syncOutput=Disabled  sampleTime=-1  eventPrescaler=0  selectMode=Continuous  enableOneShot=off  stopValue=Capture Event 2  resetEv1Ts=off  ev1Polarity=Falling Edge  resetEv2Ts=on  ev2Polarity=Rising Edge  resetEv3Ts=off  ev3Polarity=Rising Edge  resetEv4Ts=on  ev4Polarity=Rising Edge  tSCntrDataType=uint32  capEvFlag=off  capFlagDataType=uint16  overFlowFlag=off  overFlowFlagDataType=uint16  periodUnit=Seconds  periodSource=Specify via dialog  waveformPeriod=0.001  dutyUnit=Percentages  dutySource=Specify via dialog  dutyCycle=50  outputPolarity=Active High  enableCEVT1Int=off  enableCEVT2Int=on  enableCEVT3Int=off  enableCEVT4Int=on  enableCTROVFInt=off  enablePRDInt=off  enableCMPInt=off
      settings: SourceProductName=Embedded Coder Support Package for Texas Instruments C2000 Processors  SourceProductBaseCode=TIC2000
  wires:
  eCAP/1 -> MinMax/1
  MinMax/1 -> Filter Glitches/1
  Filter Glitches/1 -> Counter/Action

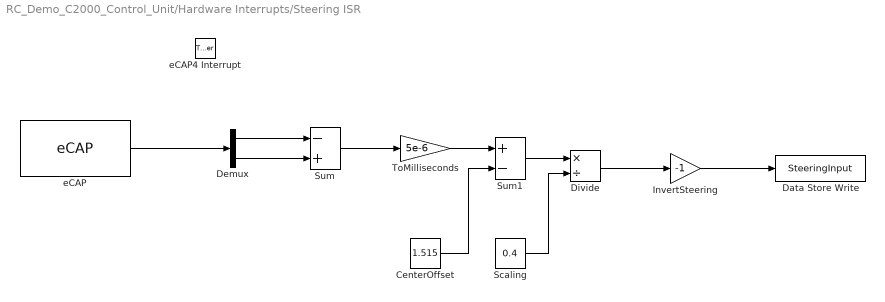
== system RC_Demo_C2000_Control_Unit/Hardware Interrupts/Steering ISR ==
  eCAP4 Interrupt : TriggerPort  TriggerType=function-call  VariantControl=Variant
  CenterOffset : Constant  Value=1.515
  Data Store Write : DataStoreWrite  DataStoreName=SteeringInput
  Demux : Demux  Outputs=2
  Divide : Product  Inputs=*/
  InvertSteering : Gain  Gain=-1
  Scaling : Constant  Value=0.4
  Sum : Sum  Inputs=-+
  Sum1 : Sum  Inputs=+-
  ToMilliseconds : Gain  Gain=5e-6  LockScale=on
  eCAP : c280xlib/eCAP  operatingMode=eCAP  selectCAPx=eCAP4  offsetValue=0  counterSynIn=off  enableCounter=off  syncOutput=Disabled  sampleTime=-1  eventPrescaler=0  selectMode=Continuous  enableOneShot=off  stopValue=Capture Event 2  resetEv1Ts=off  ev1Polarity=Rising Edge  resetEv2Ts=off  ev2Polarity=Falling Edge  resetEv3Ts=off  ev3Polarity=Rising Edge  resetEv4Ts=on  ev4Polarity=Rising Edge  tSCntrDataType=uint32  capEvFlag=off  capFlagDataType=uint16  overFlowFlag=off  overFlowFlagDataType=uint16  periodUnit=Seconds  periodSource=Specify via dialog  waveformPeriod=0.001  dutyUnit=Percentages  dutySource=Specify via dialog  dutyCycle=50  outputPolarity=Active High  enableCEVT1Int=off  enableCEVT2Int=on  enableCEVT3Int=off  enableCEVT4Int=on  enableCTROVFInt=off  enablePRDInt=off  enableCMPInt=off
      settings: SourceProductName=Embedded Coder Support Package for Texas Instruments C2000 Processors  SourceProductBaseCode=TIC2000
  wires:
  Demux/1 -> Sum/1
  Sum/1 -> ToMilliseconds/1
  eCAP/1 -> Demux/1
  CenterOffset/1 -> Sum1/2
  ToMilliseconds/1 -> Sum1/1
  Sum1/1 -> Divide/1
  Divide/1 -> InvertSteering/1
  Demux/2 -> Sum/2
  Scaling/1 -> Divide/2
  InvertSteering/1 -> Data Store Write/1

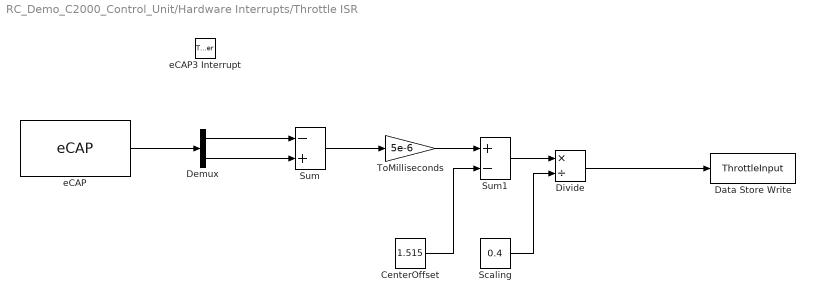
== system RC_Demo_C2000_Control_Unit/Hardware Interrupts/Throttle ISR ==
  eCAP3 Interrupt : TriggerPort  TriggerType=function-call  VariantControl=Variant
  CenterOffset : Constant  Value=1.515
  Data Store Write : DataStoreWrite  DataStoreName=ThrottleInput
  Demux : Demux  Outputs=2
  Divide : Product  Inputs=*/
  Scaling : Constant  Value=0.4
  Sum : Sum  Inputs=-+
  Sum1 : Sum  Inputs=+-
  ToMilliseconds : Gain  Gain=5e-6  LockScale=on
  eCAP : c280xlib/eCAP  operatingMode=eCAP  selectCAPx=eCAP3  offsetValue=0  counterSynIn=off  enableCounter=off  syncOutput=Disabled  sampleTime=-1  eventPrescaler=0  selectMode=Continuous  enableOneShot=off  stopValue=Capture Event 2  resetEv1Ts=off  ev1Polarity=Rising Edge  resetEv2Ts=off  ev2Polarity=Falling Edge  resetEv3Ts=off  ev3Polarity=Rising Edge  resetEv4Ts=on  ev4Polarity=Rising Edge  tSCntrDataType=uint32  capEvFlag=off  capFlagDataType=uint16  overFlowFlag=off  overFlowFlagDataType=uint16  periodUnit=Seconds  periodSource=Specify via dialog  waveformPeriod=0.001  dutyUnit=Percentages  dutySource=Specify via dialog  dutyCycle=50  outputPolarity=Active High  enableCEVT1Int=off  enableCEVT2Int=on  enableCEVT3Int=off  enableCEVT4Int=on  enableCTROVFInt=off  enablePRDInt=off  enableCMPInt=off
      settings: SourceProductName=Embedded Coder Support Package for Texas Instruments C2000 Processors  SourceProductBaseCode=TIC2000
  wires:
  Demux/1 -> Sum/1
  Sum/1 -> ToMilliseconds/1
  eCAP/1 -> Demux/1
  CenterOffset/1 -> Sum1/2
  ToMilliseconds/1 -> Sum1/1
  Sum1/1 -> Divide/1
  Demux/2 -> Sum/2
  Scaling/1 -> Divide/2
  Divide/1 -> Data Store Write/1

== system RC_Demo_C2000_Control_Unit/Hardware Interrupts/Hall Sensor A ISR/Counter ==
  Action Port : ActionPort  ActionPortLabel=if { }
  Constant : Constant  OutDataTypeStr=uint16
  Data Store Read : DataStoreRead  DataStoreName=Encoder1Counts
  Data Store Write : DataStoreWrite  DataStoreName=Encoder1Counts
  Sum1 : Sum  Inputs=|++
  wires:
  Data Store Read/1 -> Sum1/1
  Sum1/1 -> Data Store Write/1
  Constant/1 -> Sum1/2

== system RC_Demo_C2000_Control_Unit/Hardware Interrupts/Hall Sensor B ISR/Counter ==
  Action Port : ActionPort  ActionPortLabel=if { }
  Constant : Constant  OutDataTypeStr=uint16
  Data Store Read : DataStoreRead  DataStoreName=Encoder2Counts
  Data Store Write : DataStoreWrite  DataStoreName=Encoder2Counts
  Sum1 : Sum  Inputs=|++
  wires:
  Constant/1 -> Sum1/2
  Sum1/1 -> Data Store Write/1
  Data Store Read/1 -> Sum1/1
